simulink model "FlameAnalysis"  (R2015b)
settings: Solver=ode45  SolverMode=SingleTasking  StartTime=0.0  StopTime=1000  RelTol=1e-3
PreLoadFcn:
  | fprintf('loading now...\n')
PostLoadFcn:
  | model_name = gcs;
  | video_player_name=[model_name, '/From Multimedia File'];
  | video_path=get_param(video_player_name,'inputFileName');
  | model_path= get_param(model_name,'filename');
  | i=findstr('\',model_path);
  | 
  | if(~exist(video_path))
  |      video_path2=[model_path(1:i(end))  video_path(findstr('Video',video_path):end)];
  | 
  |      if(exist(video_path2))
  |           set_param(video_player_name,'inputFileName',video_path2);
  |      else
  |           j=findstr('\',video_path);
  |           video_path2=[model_path(1:i(end))  'Videos\' video_path(j(end)+1:end)];
  |           if(exist(video_path2))
  |                set_param(video_player_name,'inputFileName',video_path2);
  |           else
  |                avifiles=dir('videos\*.avi')
  |                set_param(video_player_name,'inputFileName',[model_path(1:i(end))  'Videos\'   avifiles(1).name]);
  |           end
  | 
  |      end
  | end
InitFcn:
  | clc
  | clear
  | global  t position wide dz_dt d2z_dt2 d3z_dt3 Af As dA_dt filePath Su_ Su alfa Karlovitz threshold model_name bords tWalls sheet model_path simulating numPointsAnalysis
  | simulating=true;
  | model_name = gcs;
  | model_path = [model_name, '/Edit Parameters'];
  | tbf = str2num(get_param(model_path,'tbf'));
  | ppcm= str2num(get_param(model_path,'ppcm'));
  | p2e= str2num(get_param(model_path,'p2e'));
  | 
  | nframes0= str2num(get_param(model_path,'nframes0'));
  | alfa= str2num(get_param(model_path,'alfa'));
  | fff= str2num(get_param(model_path,'fff'));
  | 
  | if((size(fff,2)~=1) & (size(fff,2)~=2))
  |     error('The flame front fraction must be scalar or 1x2-array');
  | end
  | order=str2num(get_param(model_path,'order'));
  | numberOfPoints=str2num(get_param(model_path,'numberOfPoints'));
  | orderAnalysis=str2num(get_param(model_path,'orderAnalysis'));
  | numPointsAnalysis=str2num(get_param(model_path,'numPointsAnalysis'));
  | uselog=str2num(get_param(model_path,'uselog'));
  | 
  | 
  | save2xls= strcmp('on',get_param(model_path,'save2xls'));
  | saveVideo= strcmp('on',get_param(model_path,'saveVideo'));
  | cfs= strcmp('on',get_param(model_path,'cfs'));
  | c3dv= strcmp('on',get_param(model_path,'c3dv'));
  | 
  | 
  | if(strcmp(get_param(model_path,'bge'),'Temporal Median Estimator'))
  |      bge=1;
  | elseif (strcmp(get_param(model_path,'bge'),'Temporal Median'))
  |     bge=2;
  |     bkgnd{1}=[gcs '/Background Estimator/Decomposing Red Movement/BG1/Temporal Median/Temporal Median'];
  |     bkgnd{2}=[gcs '/Background Estimator/Decomposing Green Movement/BG1/Temporal Median/Temporal Median'];
  |     bkgnd{3}=[gcs '/Background Estimator/Decomposing Blue Movement/BG1/Temporal Median/Temporal Median'];
  | 
  |     nframes0=max(nframes0,1);
  |     set_param([gcs '/Edit Parameters/'],'nframes0',num2str(nframes0));
  |     for i=1:3
  |         set_param(bkgnd{i}, 'tw', num2str(nframes0));
  |     end
  | else
  |     bge=3;
  | end
  | 
  | 
  | 
  | switch(get_param(model_path,'aprox_type'))
  |      case 'Profile'
  |            aprox_type=1;
  |            sheet='Profile';
  |      case 'Paraboloid (moving base)'
  |            aprox_type=2;
  |            sheet='Paraboloid';
  |      case 'Paraboloid(fixed base)'
  |            aprox_type=3;
  |            sheet='ParaboloidFB';
  |      case 'Spheroid'
  | ... (+19 lines)
StopFcn:
  | global editing  simulating
  | simulating = true;
  | try
  |       closeFunction
  | catch err
  |       simulating=false;
  |       err
  | end
  |   simulating=false;
model workspace (MATLAB code in the model file):
  | line_row =  22;
values from neighbouring files (symbols this model uses):
  m = size(BW,1)    [flameFront.m]    (also in putCircles.m = (y(i+1)-y(i))./(x(i+1)-x(i)))
  n = n(n==size(num,2)/4)    [averageOfVideos.m]    (also in countFramesOfVideo.m = 1; putCircles.m = length(y))
  vector = cast([row, col],'double')    [flameFront.m]
undefined symbols (not defined in the file or in its folder): strel
libraries: simulink x27, visionstatistics x14, visionconversions x9, visiontextngfix x9, visionmorphops x7, dspvision x4, visionsinks x2, visiongeotforms x1
(part 2 of 3)

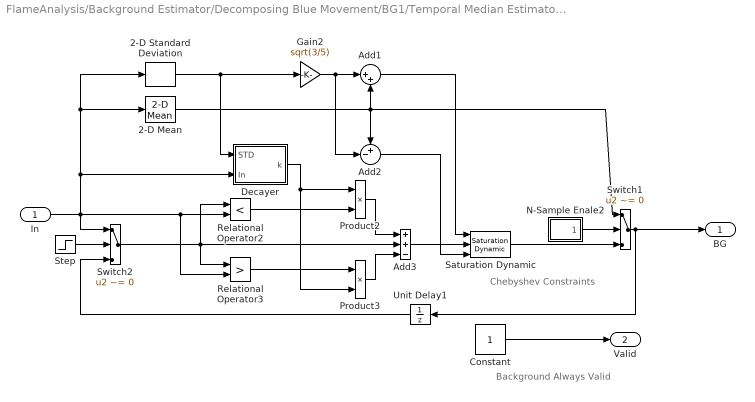
== system FlameAnalysis/Background Estimator/Decomposing Blue Movement/BG1/Temporal Median Estimator/Temporal Median Estimator ==
  note: Background
      | Always Valid
  note: Chebyshev
      | Constraints
  In : Inport
  2-D Mean : visionstatistics/2-D Mean  run=on  reset_popup=None  directionMode=Entire input  dimension=1  treatSBRowAsCol=on  roiEnable=off  roiType=Rectangles  roiPortion=Entire ROI  roiOutput=Individual statistics for each ROI  roiFlag=off  outputDataTypeStr=Inherit: Same as accumulator  outputLastDataTypeStr=Inherit: Same as accumulator  outputMin=[]  outputMax=[]  roundingMode=Floor  overflowMode=off
  2-D Standard Deviation : visionstatistics/2-D Standard Deviation  run=on  reset_popup=None  directionMode=Entire input  dimension=1  treatSBRowAsCol=on  roiEnable=off  roiType=Rectangles  roiPortion=Entire ROI  roiOutput=Individual statistics for each ROI  roiFlag=off
  Add1 : Sum  Inputs=|++
  Add2 : Sum  Inputs=+-|
  Add3 : Sum  Inputs=++-
  Constant : Constant  OutDataTypeStr=boolean
  Decayer : Subsystem
  Gain2 : Gain  Gain=sqrt(3/5)
  N-Sample Enale2 : Subsystem  mask(N Sample Enable){sample=t0}
      mask prompts: sample "Trigger Count, N"
      mask help: Active Level = Low(0)
  Product2 : Product  RndMeth=Zero
  Product3 : Product  RndMeth=Zero
  Relational Operator2 : RelationalOperator  Operator=<  OutDataTypeStr=uint(8)
  Relational Operator3 : RelationalOperator  Operator=>  OutDataTypeStr=uint(8)
  Saturation Dynamic : simulink/Discontinuities/Saturation Dynamic  OutMin=[]  OutMax=[]  OutDataTypeStr=Inherit: Same as second input  OutDataType=fixdt(1, 16)  OutScaling=2^-10  DoSatur=off
  Step : Step  Time=eps  Before=1  After=0
  Switch1 : Switch  Criteria=u2 ~= 0
  Switch2 : Switch  Criteria=u2 ~= 0
  Unit Delay1 : UnitDelay  SampleTime=-1
  BG : Outport
  Valid : Outport  Port=2
  wires:
  Add1/1 -> Saturation Dynamic/1
  Constant/1 -> Valid/1
  Add2/1 -> Saturation Dynamic/3
  2-D Mean/1 -> Add2/1, Add1/2, Switch1/1
  Gain2/1 -> Add2/2, Add1/1
  Add3/1 -> Saturation Dynamic/2
  Step/1 -> Switch2/2
  Unit Delay1/1 -> Switch2/3
  Switch2/1 -> Add3/2, Relational Operator2/1, Relational Operator3/1
  N-Sample Enale2/1(Enable) -> Switch1/2
  Switch1/1 -> BG/1, Unit Delay1/1
  In/1 -> Switch2/1, Relational Operator2/2, Relational Operator3/2, 2-D Standard Deviation/1, 2-D Mean/1, Decayer/2(In)
  Relational Operator2/1 -> Product2/2
  Relational Operator3/1 -> Product3/1
  Saturation Dynamic/1 -> Switch1/3
  2-D Standard Deviation/1 -> Decayer/1(STD), Gain2/1
  Decayer/1(k) -> Product2/1, Product3/2
  Product2/1 -> Add3/1
  Product3/1 -> Add3/3

== system FlameAnalysis/Background Estimator/Decomposing Green Movement/BG1/Motion Based Background Estimator/Motion Based Background Estimator ==
  In : Inport
  BG_running : Subsystem
  Logical Operator : Logic  Operator=NOT
  Unit Delay : UnitDelay  SampleTime=-1
  BG : Outport
  Valid : Outport  Port=2
  wires:
  Unit Delay/1 -> Logical Operator/1
  BG_running/1(BG) -> BG/1
  In/1 -> BG_running/1(In1)
  Logical Operator/1 -> BG_running/Enable
  BG_running/2(bgflag) -> Valid/1, Unit Delay/1

== system FlameAnalysis/Background Estimator/Decomposing Green Movement/BG1/Temporal Median/Temporal Median ==
  In : Inport
  Background estimator : Subsystem  TreatAsAtomicUnit=on
  Logical Operator1 : Logic  Operator=NOT
  N-Sample Enale2 : Subsystem  mask(N Sample Enable){sample=tw}
      mask prompts: sample "Trigger Count, N"
      mask help: Active Level = Low(0)
  BG : Outport
  Valid : Outport  Port=2
  wires:
  In/1 -> Background estimator/1(Video In)
  Background estimator/1(Background) -> BG/1
  N-Sample Enale2/1(Enable) -> Background estimator/Enable, Logical Operator1/1
  Logical Operator1/1 -> Valid/1

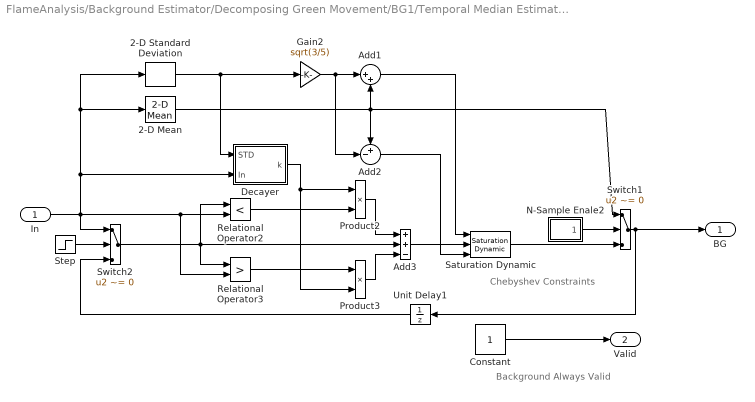
== system FlameAnalysis/Background Estimator/Decomposing Green Movement/BG1/Temporal Median Estimator/Temporal Median Estimator ==
  note: Background
      | Always Valid
  note: Chebyshev
      | Constraints
  In : Inport
  2-D Mean : visionstatistics/2-D Mean  run=on  reset_popup=None  directionMode=Entire input  dimension=1  treatSBRowAsCol=on  roiEnable=off  roiType=Rectangles  roiPortion=Entire ROI  roiOutput=Individual statistics for each ROI  roiFlag=off  outputDataTypeStr=Inherit: Same as accumulator  outputLastDataTypeStr=Inherit: Same as accumulator  outputMin=[]  outputMax=[]  roundingMode=Floor  overflowMode=off
  2-D Standard Deviation : visionstatistics/2-D Standard Deviation  run=on  reset_popup=None  directionMode=Entire input  dimension=1  treatSBRowAsCol=on  roiEnable=off  roiType=Rectangles  roiPortion=Entire ROI  roiOutput=Individual statistics for each ROI  roiFlag=off
  Add1 : Sum  Inputs=|++
  Add2 : Sum  Inputs=+-|
  Add3 : Sum  Inputs=++-
  Constant : Constant  OutDataTypeStr=boolean
  Decayer : Subsystem
  Gain2 : Gain  Gain=sqrt(3/5)
  N-Sample Enale2 : Subsystem  mask(N Sample Enable){sample=t0}
      mask prompts: sample "Trigger Count, N"
      mask help: Active Level = Low(0)
  Product2 : Product  RndMeth=Zero
  Product3 : Product  RndMeth=Zero
  Relational Operator2 : RelationalOperator  Operator=<  OutDataTypeStr=uint(8)
  Relational Operator3 : RelationalOperator  Operator=>  OutDataTypeStr=uint(8)
  Saturation Dynamic : simulink/Discontinuities/Saturation Dynamic  OutMin=[]  OutMax=[]  OutDataTypeStr=Inherit: Same as second input  OutDataType=fixdt(1, 16)  OutScaling=2^-10  DoSatur=off
  Step : Step  Time=eps  Before=1  After=0
  Switch1 : Switch  Criteria=u2 ~= 0
  Switch2 : Switch  Criteria=u2 ~= 0
  Unit Delay1 : UnitDelay  SampleTime=-1
  BG : Outport
  Valid : Outport  Port=2
  wires:
  Add1/1 -> Saturation Dynamic/1
  Constant/1 -> Valid/1
  Add2/1 -> Saturation Dynamic/3
  2-D Mean/1 -> Add2/1, Add1/2, Switch1/1
  Gain2/1 -> Add2/2, Add1/1
  Add3/1 -> Saturation Dynamic/2
  Step/1 -> Switch2/2
  Unit Delay1/1 -> Switch2/3
  Switch2/1 -> Add3/2, Relational Operator2/1, Relational Operator3/1
  N-Sample Enale2/1(Enable) -> Switch1/2
  Switch1/1 -> BG/1, Unit Delay1/1
  In/1 -> Switch2/1, Relational Operator2/2, Relational Operator3/2, 2-D Standard Deviation/1, 2-D Mean/1, Decayer/2(In)
  Relational Operator2/1 -> Product2/2
  Relational Operator3/1 -> Product3/1
  Saturation Dynamic/1 -> Switch1/3
  2-D Standard Deviation/1 -> Decayer/1(STD), Gain2/1
  Decayer/1(k) -> Product2/1, Product3/2
  Product2/1 -> Add3/1
  Product3/1 -> Add3/3

== system FlameAnalysis/Background Estimator/Decomposing Red Movement/BG1/Motion Based Background Estimator/Motion Based Background Estimator ==
  In : Inport
  BG_running : Subsystem
  Logical Operator : Logic  Operator=NOT
  Unit Delay : UnitDelay  SampleTime=-1
  BG : Outport
  Valid : Outport  Port=2
  wires:
  Unit Delay/1 -> Logical Operator/1
  BG_running/1(BG) -> BG/1
  In/1 -> BG_running/1(In1)
  Logical Operator/1 -> BG_running/Enable
  BG_running/2(bgflag) -> Valid/1, Unit Delay/1

== system FlameAnalysis/Background Estimator/Decomposing Red Movement/BG1/Temporal Median/Temporal Median ==
  In : Inport
  Background estimator : Subsystem  TreatAsAtomicUnit=on
  Logical Operator1 : Logic  Operator=NOT
  N-Sample Enale2 : Subsystem  mask(N Sample Enable){sample=tw}
      mask prompts: sample "Trigger Count, N"
      mask help: Active Level = Low(0)
  BG : Outport
  Valid : Outport  Port=2
  wires:
  In/1 -> Background estimator/1(Video In)
  Background estimator/1(Background) -> BG/1
  N-Sample Enale2/1(Enable) -> Background estimator/Enable, Logical Operator1/1
  Logical Operator1/1 -> Valid/1

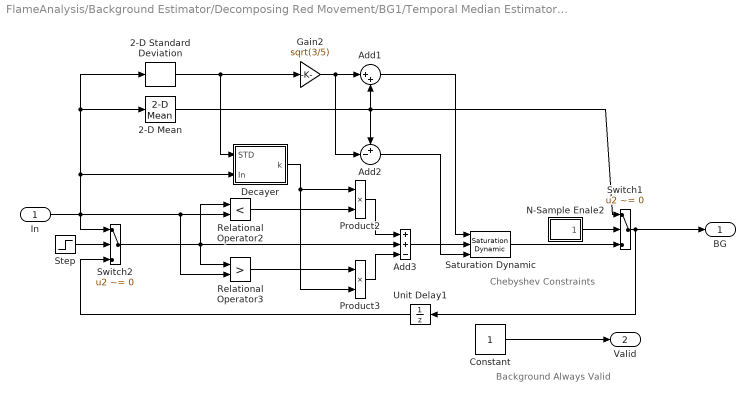
== system FlameAnalysis/Background Estimator/Decomposing Red Movement/BG1/Temporal Median Estimator/Temporal Median Estimator ==
  note: Background
      | Always Valid
  note: Chebyshev
      | Constraints
  In : Inport
  2-D Mean : visionstatistics/2-D Mean  run=on  reset_popup=None  directionMode=Entire input  dimension=1  treatSBRowAsCol=on  roiEnable=off  roiType=Rectangles  roiPortion=Entire ROI  roiOutput=Individual statistics for each ROI  roiFlag=off  outputDataTypeStr=Inherit: Same as accumulator  outputLastDataTypeStr=Inherit: Same as accumulator  outputMin=[]  outputMax=[]  roundingMode=Floor  overflowMode=off
  2-D Standard Deviation : visionstatistics/2-D Standard Deviation  run=on  reset_popup=None  directionMode=Entire input  dimension=1  treatSBRowAsCol=on  roiEnable=off  roiType=Rectangles  roiPortion=Entire ROI  roiOutput=Individual statistics for each ROI  roiFlag=off
  Add1 : Sum  Inputs=|++
  Add2 : Sum  Inputs=+-|
  Add3 : Sum  Inputs=++-
  Constant : Constant  OutDataTypeStr=boolean
  Decayer : Subsystem
  Gain2 : Gain  Gain=sqrt(3/5)
  N-Sample Enale2 : Subsystem  mask(N Sample Enable){sample=t0}
      mask prompts: sample "Trigger Count, N"
      mask help: Active Level = Low(0)
  Product2 : Product  RndMeth=Zero
  Product3 : Product  RndMeth=Zero
  Relational Operator2 : RelationalOperator  Operator=<  OutDataTypeStr=uint(8)
  Relational Operator3 : RelationalOperator  Operator=>  OutDataTypeStr=uint(8)
  Saturation Dynamic : simulink/Discontinuities/Saturation Dynamic  OutMin=[]  OutMax=[]  OutDataTypeStr=Inherit: Same as second input  OutDataType=fixdt(1, 16)  OutScaling=2^-10  DoSatur=off
  Step : Step  Time=eps  Before=1  After=0
  Switch1 : Switch  Criteria=u2 ~= 0
  Switch2 : Switch  Criteria=u2 ~= 0
  Unit Delay1 : UnitDelay  SampleTime=-1
  BG : Outport
  Valid : Outport  Port=2
  wires:
  Add1/1 -> Saturation Dynamic/1
  Constant/1 -> Valid/1
  Add2/1 -> Saturation Dynamic/3
  2-D Mean/1 -> Add2/1, Add1/2, Switch1/1
  Gain2/1 -> Add2/2, Add1/1
  Add3/1 -> Saturation Dynamic/2
  Step/1 -> Switch2/2
  Unit Delay1/1 -> Switch2/3
  Switch2/1 -> Add3/2, Relational Operator2/1, Relational Operator3/1
  N-Sample Enale2/1(Enable) -> Switch1/2
  Switch1/1 -> BG/1, Unit Delay1/1
  In/1 -> Switch2/1, Relational Operator2/2, Relational Operator3/2, 2-D Standard Deviation/1, 2-D Mean/1, Decayer/2(In)
  Relational Operator2/1 -> Product2/2
  Relational Operator3/1 -> Product3/1
  Saturation Dynamic/1 -> Switch1/3
  2-D Standard Deviation/1 -> Decayer/1(STD), Gain2/1
  Decayer/1(k) -> Product2/1, Product3/2
  Product2/1 -> Add3/1
  Product3/1 -> Add3/3

== system FlameAnalysis/Background Estimator/Decomposing Blue Movement/BG1/Motion Based Background Estimator/Motion Based Background Estimator/BG_running ==
  In1 : Inport
  Enable : EnablePort  PropagateVarSize=During execution
  CompleteBG : Subsystem
  Compositing : visiontextngfix/Compositing  operation=Binary mask  bFacSrc=Specify via dialog  mFacSrc=Input port  bFactor=0.75  mFactor=1  source=Specify via dialog  coordinates=[1 1]  prodOutputMode=Binary point scaling  prodOutputWordLength=32  prodOutputFracLength=10  roundingMode=Floor  overflowMode=off
  EvaluateFG : Subsystem
  N-Sample Enable3 : Subsystem  mask(N-Sample Enable){sample=2}
      mask prompts: sample "Trigger Count, N"
      mask help: Active = High(0)
  Switch : Switch  Criteria=u2 ~= 0
  Unit Delay : UnitDelay  SampleTime=-1
  BG : Outport
  bgflag : Outport  Port=2
  wires:
  Compositing/1 -> BG/1, Switch/1
  CompleteBG/1(fgmask) -> Compositing/3
  EvaluateFG/1(fgB) -> CompleteBG/1(fgB)
  In1/1 -> EvaluateFG/1(I), Compositing/2, Switch/3
  CompleteBG/2(bgflag) -> bgflag/1
  N-Sample Enable3/1(Enable) -> Switch/2
  Switch/1 -> Unit Delay/1
  Unit Delay/1 -> Compositing/1

== system FlameAnalysis/Background Estimator/Decomposing Blue Movement/BG1/Temporal Median/Temporal Median/Background estimator ==
  note: Estimate the background
  Video In : Inport
  Enable : EnablePort  PropagateVarSize=During execution
  2-D Median : visionstatistics/2-D Median  sortAlg=Quick sort  directionMode=Each column  dimension=1  treatSBRowAsCol=on  outputDataTypeStr=Inherit: Same as accumulator  outputLastDataTypeStr=Inherit: Same as accumulator  outputMin=[]  outputMax=[]  accumDataTypeStr=Inherit: Same as product output  accumLastDataTypeStr=Inherit: Same as product output  roundingMode=Floor  overflowMode=off
      settings: allowOverrides=off
  Buffer : Buffer  N=tw  V=tw-1  TreatMby1Signals=One channel
  Frame Conversion1 : FrameConversion  InheritSamplingMode=off  OutFrame=Sample-based
  Reshape : Reshape  OutputDimensionality=Row vector (2-D)
  Reshape1 : Reshape  OutputDimensionality=Derive from reference input port  OutputDimensions=[120 160]
  Background : Outport
  wires:
  Reshape1/1 -> Background/1
  Reshape/1 -> Buffer/1
  Video In/1 -> Reshape/1, Reshape1/2
  Frame Conversion1/1 -> Reshape1/1
  Buffer/1 -> 2-D Median/1
  2-D Median/1 -> Frame Conversion1/1

== system FlameAnalysis/Background Estimator/Decomposing Blue Movement/BG1/Temporal Median/Temporal Median/N-Sample Enale2 ==
  Constant : Constant  OutDataTypeStr=boolean
  Constant1 : Constant  Value=0  OutDataTypeStr=boolean
  Counter Limited : simulink/Sources/Counter Limited  uplimit=sample  tsamp=-1
  Enabled Subsystem : Subsystem  TreatAsAtomicUnit=on
  Switch : Switch  Threshold=sample
  Enable : Outport
  wires:
  Enabled Subsystem/1(Out1) -> Enable/1
  Switch/1 -> Enabled Subsystem/Enable
  Constant/1 -> Switch/1
  Constant1/1 -> Switch/3
  Counter Limited/1 -> Switch/2

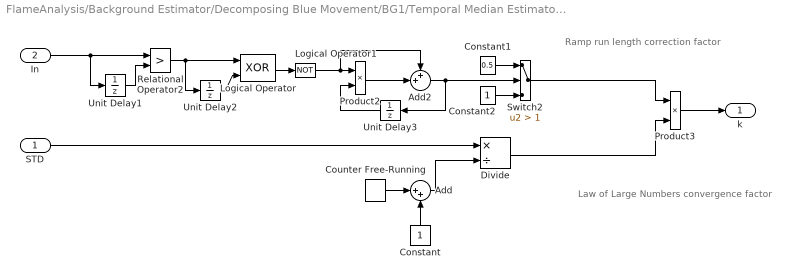
== system FlameAnalysis/Background Estimator/Decomposing Blue Movement/BG1/Temporal Median Estimator/Temporal Median Estimator/Decayer ==
  note: Ramp run length correction factor
  note: Law of Large Numbers convergence factor
  STD : Inport
  In : Inport  Port=2
  Add : Sum  Inputs=|++
  Add2 : Sum  Inputs=++|  OutDataTypeStr=single
  Constant : Constant  OutDataTypeStr=single
  Constant1 : Constant  Value=0.5  OutDataTypeStr=Inherit: Inherit via back propagation
  Constant2 : Constant  OutDataTypeStr=Inherit: Inherit via back propagation
  Counter Free-Running : simulink/Sources/Counter Free-Running  NumBits=16  tsamp=-1
  Divide : Product  Inputs=*/  OutDataTypeStr=single
  Logical Operator : Logic  Operator=XOR  AllPortsSameDT=off  OutDataTypeStr=boolean
  Logical Operator1 : Logic  Operator=NOT  AllPortsSameDT=off  OutDataTypeStr=boolean
  Product2 : Product  RndMeth=Zero
  Product3 : Product  RndMeth=Zero
  Relational Operator2 : RelationalOperator  Operator=>  OutDataTypeStr=boolean
  Switch2 : Switch  Criteria=u2 > Threshold  Threshold=1
  Unit Delay1 : UnitDelay  SampleTime=-1
  Unit Delay2 : UnitDelay  InitialCondition=1  SampleTime=-1
  Unit Delay3 : UnitDelay  SampleTime=-1
  k : Outport
  wires:
  Constant/1 -> Add/2
  Constant1/1 -> Switch2/1
  Constant2/1 -> Switch2/3
  Product3/1 -> k/1
  In/1 -> Unit Delay1/1, Relational Operator2/1
  Unit Delay3/1 -> Product2/2
  Add2/1 -> Switch2/2, Unit Delay3/1
  Product2/1 -> Add2/2
  Logical Operator1/1 -> Product2/1, Add2/1
  Logical Operator/1 -> Logical Operator1/1
  Unit Delay2/1 -> Logical Operator/2
  Relational Operator2/1 -> Unit Delay2/1, Logical Operator/1
  Unit Delay1/1 -> Relational Operator2/2
  STD/1 -> Divide/1
  Counter Free-Running/1 -> Add/1
  Add/1 -> Divide/2
  Divide/1 -> Product3/2
  Switch2/1 -> Product3/1

== system FlameAnalysis/Background Estimator/Decomposing Blue Movement/BG1/Temporal Median Estimator/Temporal Median Estimator/N-Sample Enale2 ==
  Constant : Constant  OutDataTypeStr=boolean
  Constant1 : Constant  Value=0  OutDataTypeStr=boolean
  Counter Limited : simulink/Sources/Counter Limited  uplimit=sample  tsamp=-1
  Enabled Subsystem : Subsystem  TreatAsAtomicUnit=on
  Switch : Switch  Threshold=sample
  Enable : Outport
  wires:
  Enabled Subsystem/1(Out1) -> Enable/1
  Switch/1 -> Enabled Subsystem/Enable
  Constant/1 -> Switch/1
  Constant1/1 -> Switch/3
  Counter Limited/1 -> Switch/2

== system FlameAnalysis/Background Estimator/Decomposing Green Movement/BG1/Motion Based Background Estimator/Motion Based Background Estimator/BG_running ==
  In1 : Inport
  Enable : EnablePort  PropagateVarSize=During execution
  CompleteBG : Subsystem
  Compositing : visiontextngfix/Compositing  operation=Binary mask  bFacSrc=Specify via dialog  mFacSrc=Input port  bFactor=0.75  mFactor=1  source=Specify via dialog  coordinates=[1 1]  prodOutputMode=Binary point scaling  prodOutputWordLength=32  prodOutputFracLength=10  roundingMode=Floor  overflowMode=off
  EvaluateFG : Subsystem
  N-Sample Enable3 : Subsystem  mask(N-Sample Enable){sample=2}
      mask prompts: sample "Trigger Count, N"
      mask help: Active = High(0)
  Switch : Switch  Criteria=u2 ~= 0
  Unit Delay : UnitDelay  SampleTime=-1
  BG : Outport
  bgflag : Outport  Port=2
  wires:
  Compositing/1 -> BG/1, Switch/1
  CompleteBG/1(fgmask) -> Compositing/3
  EvaluateFG/1(fgB) -> CompleteBG/1(fgB)
  In1/1 -> EvaluateFG/1(I), Compositing/2, Switch/3
  CompleteBG/2(bgflag) -> bgflag/1
  N-Sample Enable3/1(Enable) -> Switch/2
  Switch/1 -> Unit Delay/1
  Unit Delay/1 -> Compositing/1

== system FlameAnalysis/Background Estimator/Decomposing Green Movement/BG1/Temporal Median/Temporal Median/Background estimator ==
  note: Estimate the background
  Video In : Inport
  Enable : EnablePort  PropagateVarSize=During execution
  2-D Median : visionstatistics/2-D Median  sortAlg=Quick sort  directionMode=Each column  dimension=1  treatSBRowAsCol=on  outputDataTypeStr=Inherit: Same as accumulator  outputLastDataTypeStr=Inherit: Same as accumulator  outputMin=[]  outputMax=[]  accumDataTypeStr=Inherit: Same as product output  accumLastDataTypeStr=Inherit: Same as product output  roundingMode=Floor  overflowMode=off
      settings: allowOverrides=off
  Buffer : Buffer  N=tw  V=tw-1  TreatMby1Signals=One channel
  Frame Conversion1 : FrameConversion  InheritSamplingMode=off  OutFrame=Sample-based
  Reshape : Reshape  OutputDimensionality=Row vector (2-D)
  Reshape1 : Reshape  OutputDimensionality=Derive from reference input port  OutputDimensions=[120 160]
  Background : Outport
  wires:
  Reshape1/1 -> Background/1
  Reshape/1 -> Buffer/1
  Video In/1 -> Reshape/1, Reshape1/2
  Frame Conversion1/1 -> Reshape1/1
  Buffer/1 -> 2-D Median/1
  2-D Median/1 -> Frame Conversion1/1

== system FlameAnalysis/Background Estimator/Decomposing Green Movement/BG1/Temporal Median/Temporal Median/N-Sample Enale2 ==
  Constant : Constant  OutDataTypeStr=boolean
  Constant1 : Constant  Value=0  OutDataTypeStr=boolean
  Counter Limited : simulink/Sources/Counter Limited  uplimit=sample  tsamp=-1
  Enabled Subsystem : Subsystem  TreatAsAtomicUnit=on
  Switch : Switch  Threshold=sample
  Enable : Outport
  wires:
  Enabled Subsystem/1(Out1) -> Enable/1
  Switch/1 -> Enabled Subsystem/Enable
  Constant/1 -> Switch/1
  Constant1/1 -> Switch/3
  Counter Limited/1 -> Switch/2

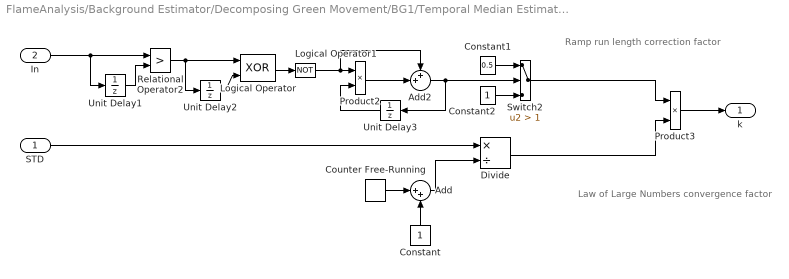
== system FlameAnalysis/Background Estimator/Decomposing Green Movement/BG1/Temporal Median Estimator/Temporal Median Estimator/Decayer ==
  note: Ramp run length correction factor
  note: Law of Large Numbers convergence factor
  STD : Inport
  In : Inport  Port=2
  Add : Sum  Inputs=|++
  Add2 : Sum  Inputs=++|  OutDataTypeStr=single
  Constant : Constant  OutDataTypeStr=single
  Constant1 : Constant  Value=0.5  OutDataTypeStr=Inherit: Inherit via back propagation
  Constant2 : Constant  OutDataTypeStr=Inherit: Inherit via back propagation
  Counter Free-Running : simulink/Sources/Counter Free-Running  NumBits=16  tsamp=-1
  Divide : Product  Inputs=*/  OutDataTypeStr=single
  Logical Operator : Logic  Operator=XOR  AllPortsSameDT=off  OutDataTypeStr=boolean
  Logical Operator1 : Logic  Operator=NOT  AllPortsSameDT=off  OutDataTypeStr=boolean
  Product2 : Product  RndMeth=Zero
  Product3 : Product  RndMeth=Zero
  Relational Operator2 : RelationalOperator  Operator=>  OutDataTypeStr=boolean
  Switch2 : Switch  Criteria=u2 > Threshold  Threshold=1
  Unit Delay1 : UnitDelay  SampleTime=-1
  Unit Delay2 : UnitDelay  InitialCondition=1  SampleTime=-1
  Unit Delay3 : UnitDelay  SampleTime=-1
  k : Outport
  wires:
  Constant/1 -> Add/2
  Constant1/1 -> Switch2/1
  Constant2/1 -> Switch2/3
  Product3/1 -> k/1
  In/1 -> Unit Delay1/1, Relational Operator2/1
  Unit Delay3/1 -> Product2/2
  Add2/1 -> Switch2/2, Unit Delay3/1
  Product2/1 -> Add2/2
  Logical Operator1/1 -> Product2/1, Add2/1
  Logical Operator/1 -> Logical Operator1/1
  Unit Delay2/1 -> Logical Operator/2
  Relational Operator2/1 -> Unit Delay2/1, Logical Operator/1
  Unit Delay1/1 -> Relational Operator2/2
  STD/1 -> Divide/1
  Counter Free-Running/1 -> Add/1
  Add/1 -> Divide/2
  Divide/1 -> Product3/2
  Switch2/1 -> Product3/1

== system FlameAnalysis/Background Estimator/Decomposing Green Movement/BG1/Temporal Median Estimator/Temporal Median Estimator/N-Sample Enale2 ==
  Constant : Constant  OutDataTypeStr=boolean
  Constant1 : Constant  Value=0  OutDataTypeStr=boolean
  Counter Limited : simulink/Sources/Counter Limited  uplimit=sample  tsamp=-1
  Enabled Subsystem : Subsystem  TreatAsAtomicUnit=on
  Switch : Switch  Threshold=sample
  Enable : Outport
  wires:
  Enabled Subsystem/1(Out1) -> Enable/1
  Switch/1 -> Enabled Subsystem/Enable
  Constant/1 -> Switch/1
  Constant1/1 -> Switch/3
  Counter Limited/1 -> Switch/2

== system FlameAnalysis/Background Estimator/Decomposing Red Movement/BG1/Motion Based Background Estimator/Motion Based Background Estimator/BG_running ==
  In1 : Inport
  Enable : EnablePort  PropagateVarSize=During execution
  CompleteBG : Subsystem
  Compositing : visiontextngfix/Compositing  operation=Binary mask  bFacSrc=Specify via dialog  mFacSrc=Input port  bFactor=0.75  mFactor=1  source=Specify via dialog  coordinates=[1 1]  prodOutputMode=Binary point scaling  prodOutputWordLength=32  prodOutputFracLength=10  roundingMode=Floor  overflowMode=off
  EvaluateFG : Subsystem
  N-Sample Enable3 : Subsystem  mask(N-Sample Enable){sample=2}
      mask prompts: sample "Trigger Count, N"
      mask help: Active = High(0)
  Switch : Switch  Criteria=u2 ~= 0
  Unit Delay : UnitDelay  SampleTime=-1
  BG : Outport
  bgflag : Outport  Port=2
  wires:
  Compositing/1 -> BG/1, Switch/1
  CompleteBG/1(fgmask) -> Compositing/3
  EvaluateFG/1(fgB) -> CompleteBG/1(fgB)
  In1/1 -> EvaluateFG/1(I), Compositing/2, Switch/3
  CompleteBG/2(bgflag) -> bgflag/1
  N-Sample Enable3/1(Enable) -> Switch/2
  Switch/1 -> Unit Delay/1
  Unit Delay/1 -> Compositing/1

== system FlameAnalysis/Background Estimator/Decomposing Red Movement/BG1/Temporal Median/Temporal Median/Background estimator ==
  note: Estimate the background
  Video In : Inport
  Enable : EnablePort  PropagateVarSize=During execution
  2-D Median : visionstatistics/2-D Median  sortAlg=Quick sort  directionMode=Each column  dimension=1  treatSBRowAsCol=on  outputDataTypeStr=Inherit: Same as accumulator  outputLastDataTypeStr=Inherit: Same as accumulator  outputMin=[]  outputMax=[]  accumDataTypeStr=Inherit: Same as product output  accumLastDataTypeStr=Inherit: Same as product output  roundingMode=Floor  overflowMode=off
      settings: allowOverrides=off
  Buffer : Buffer  N=tw  V=tw-1  TreatMby1Signals=One channel
  Frame Conversion1 : FrameConversion  InheritSamplingMode=off  OutFrame=Sample-based
  Reshape : Reshape  OutputDimensionality=Row vector (2-D)
  Reshape1 : Reshape  OutputDimensionality=Derive from reference input port  OutputDimensions=[120 160]
  Background : Outport
  wires:
  Reshape1/1 -> Background/1
  Reshape/1 -> Buffer/1
  Video In/1 -> Reshape/1, Reshape1/2
  Frame Conversion1/1 -> Reshape1/1
  Buffer/1 -> 2-D Median/1
  2-D Median/1 -> Frame Conversion1/1

== system FlameAnalysis/Background Estimator/Decomposing Red Movement/BG1/Temporal Median/Temporal Median/N-Sample Enale2 ==
  Constant : Constant  OutDataTypeStr=boolean
  Constant1 : Constant  Value=0  OutDataTypeStr=boolean
  Counter Limited : simulink/Sources/Counter Limited  uplimit=sample  tsamp=-1
  Enabled Subsystem : Subsystem  TreatAsAtomicUnit=on
  Switch : Switch  Threshold=sample
  Enable : Outport
  wires:
  Enabled Subsystem/1(Out1) -> Enable/1
  Switch/1 -> Enabled Subsystem/Enable
  Constant/1 -> Switch/1
  Constant1/1 -> Switch/3
  Counter Limited/1 -> Switch/2

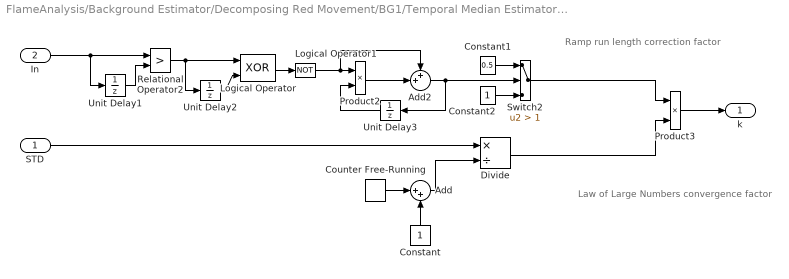
== system FlameAnalysis/Background Estimator/Decomposing Red Movement/BG1/Temporal Median Estimator/Temporal Median Estimator/Decayer ==
  note: Ramp run length correction factor
  note: Law of Large Numbers convergence factor
  STD : Inport
  In : Inport  Port=2
  Add : Sum  Inputs=|++
  Add2 : Sum  Inputs=++|  OutDataTypeStr=single
  Constant : Constant  OutDataTypeStr=single
  Constant1 : Constant  Value=0.5  OutDataTypeStr=Inherit: Inherit via back propagation
  Constant2 : Constant  OutDataTypeStr=Inherit: Inherit via back propagation
  Counter Free-Running : simulink/Sources/Counter Free-Running  NumBits=16  tsamp=-1
  Divide : Product  Inputs=*/  OutDataTypeStr=single
  Logical Operator : Logic  Operator=XOR  AllPortsSameDT=off  OutDataTypeStr=boolean
  Logical Operator1 : Logic  Operator=NOT  AllPortsSameDT=off  OutDataTypeStr=boolean
  Product2 : Product  RndMeth=Zero
  Product3 : Product  RndMeth=Zero
  Relational Operator2 : RelationalOperator  Operator=>  OutDataTypeStr=boolean
  Switch2 : Switch  Criteria=u2 > Threshold  Threshold=1
  Unit Delay1 : UnitDelay  SampleTime=-1
  Unit Delay2 : UnitDelay  InitialCondition=1  SampleTime=-1
  Unit Delay3 : UnitDelay  SampleTime=-1
  k : Outport
  wires:
  Constant/1 -> Add/2
  Constant1/1 -> Switch2/1
  Constant2/1 -> Switch2/3
  Product3/1 -> k/1
  In/1 -> Unit Delay1/1, Relational Operator2/1
  Unit Delay3/1 -> Product2/2
  Add2/1 -> Switch2/2, Unit Delay3/1
  Product2/1 -> Add2/2
  Logical Operator1/1 -> Product2/1, Add2/1
  Logical Operator/1 -> Logical Operator1/1
  Unit Delay2/1 -> Logical Operator/2
  Relational Operator2/1 -> Unit Delay2/1, Logical Operator/1
  Unit Delay1/1 -> Relational Operator2/2
  STD/1 -> Divide/1
  Counter Free-Running/1 -> Add/1
  Add/1 -> Divide/2
  Divide/1 -> Product3/2
  Switch2/1 -> Product3/1

== system FlameAnalysis/Background Estimator/Decomposing Red Movement/BG1/Temporal Median Estimator/Temporal Median Estimator/N-Sample Enale2 ==
  Constant : Constant  OutDataTypeStr=boolean
  Constant1 : Constant  Value=0  OutDataTypeStr=boolean
  Counter Limited : simulink/Sources/Counter Limited  uplimit=sample  tsamp=-1
  Enabled Subsystem : Subsystem  TreatAsAtomicUnit=on
  Switch : Switch  Threshold=sample
  Enable : Outport
  wires:
  Enabled Subsystem/1(Out1) -> Enable/1
  Switch/1 -> Enabled Subsystem/Enable
  Constant/1 -> Switch/1
  Constant1/1 -> Switch/3
  Counter Limited/1 -> Switch/2

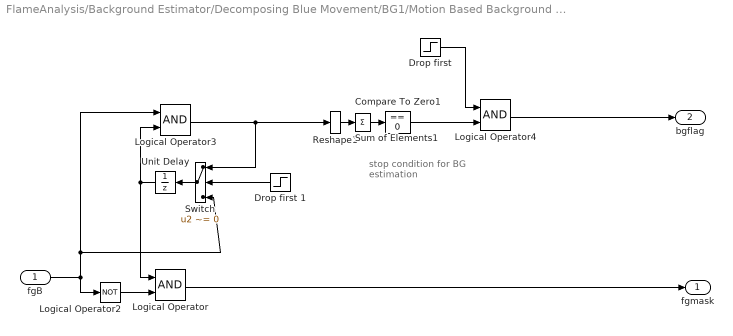
== system FlameAnalysis/Background Estimator/Decomposing Blue Movement/BG1/Motion Based Background Estimator/Motion Based Background Estimator/BG_running/CompleteBG ==
  note: stop condition
      | for BG estimation
  fgB : Inport
  Compare To Zero1 : simulink/Logic and Bit Operations/Compare To Zero  relop===  OutDataTypeStr=uint8  ZeroCross=off
  Drop first : Step  Time=eps
  Drop first 1 : Step  Time=eps
  Logical Operator : Logic  AllPortsSameDT=off  OutDataTypeStr=boolean
  Logical Operator2 : Logic  Operator=NOT  AllPortsSameDT=off  OutDataTypeStr=boolean
  Logical Operator3 : Logic  AllPortsSameDT=off  OutDataTypeStr=boolean
  Logical Operator4 : Logic  AllPortsSameDT=off  OutDataTypeStr=boolean
  Reshape1 : Reshape
  Sum of Elements1 : Sum  Inputs=+
  Switch : Switch  Criteria=u2 ~= 0
  Unit Delay : UnitDelay  SampleTime=-1
  fgmask : Outport
  bgflag : Outport  Port=2
  wires:
  fgB/1 -> Switch/3, Logical Operator3/1, Logical Operator2/1
  Logical Operator/1 -> fgmask/1
  Drop first 1/1 -> Switch/2
  Switch/1 -> Unit Delay/1
  Unit Delay/1 -> Logical Operator/1, Logical Operator3/2
  Compare To Zero1/1 -> Logical Operator4/2
  Logical Operator4/1 -> bgflag/1
  Drop first/1 -> Logical Operator4/1
  Sum of Elements1/1 -> Compare To Zero1/1
  Logical Operator3/1 -> Reshape1/1, Switch/1
  Reshape1/1 -> Sum of Elements1/1
  Logical Operator2/1 -> Logical Operator/2

== system FlameAnalysis/Background Estimator/Decomposing Blue Movement/BG1/Motion Based Background Estimator/Motion Based Background Estimator/BG_running/EvaluateFG ==
  note: detect motion for foreground
  I : Inport
  Abs3 : Abs  SaturateOnIntegerOverflow=on
  Add : Sum  Inputs=+-
  Autothreshold1 : visionconversions/Autothreshold  operator=>  threshOut=off  effMetricOut=off  userDefinedRange=off  umin=0  umax=255  outOfRngOpt=Warn and saturate  scaleThreshold=off  scaleFactor=1  P1Mode=Specify word length  P1WordLength=32  P1FracLength=30  P2Mode=Specify word length  P2WordLength=32  P2FracLength=22  P3Mode=Specify word length  P3WordLength=32  P3FracLength=14  P4Mode=Binary point scaling  P4WordLength=32  P4FracLength=15  Q1Mode=Specify word length  Q1WordLength=32  Q1FracLength=16  EMMode=Specify word length  EMWordLength=16  EMFracLength=14  roundingMode=Floor  overflowMode=off
  Blob Analysis : visionstatistics/Blob Analysis  Tag=vipblks_row_conv  area=off  centroid=off  bBox=on  majorAxis=off  minorAxis=off  angle=off  eccentricity=off  equivDiameterSq=off  extent=off  perimeter=off  maxBlobs=50  warnIfNumBlobsExceeded=on  isCount=off  useMinArea=off  minArea=0  useMaxArea=off  maxArea=inf  excludeBorderBlob=off  outDT=double  isOutVarDim=off  isFill=on  fillValues=-1  conn=8  isLabel=off  outputMode=Binary point scaling  outputWordLength=32  outputFracLength=16  firstCoeffMode=Binary point scaling  firstCoeffWordLength=16  firstCoeffFracLength=14  secondCoeffMode=Binary point scaling  secondCoeffWordLength=32  secondCoeffFracLength=16  accumMode=Binary point scaling  accumWordLength=32  accumFracLength=0  prodOutputMode=Binary point scaling  prodOutputWordLength=32  prodOutputFracLength=16  roundingMode=Floor  overflowMode=off
  BoxForeground : visiontextngfix/Draw Shapes  shape=Rectangles  fill=on  lineWidth=1  fillClrSource=Specify via dialog  display=White  intensity=200  color=[0 1 0]  opacity=1  viewport=Entire image  antialiasing=off  inType=Intensity  imagePorts=One multidimensional signal  prodOutputMode=Binary point scaling  prodOutputWordLength=32  prodOutputFracLength=14  memoryMode=Specify word length  memoryWordLength=16  memoryFracLength=15  roundingMode=Floor  overflowMode=off
  Closing : visionmorphops/Closing  nhoodsrc=Specify via dialog  strel=strel('square',5)
  Dilation : visionmorphops/Dilation  nhoodsrc=Specify via dialog  strel=[1 1 1; 1 1 1; 1 1 1]
  Manual Switch : ManualSwitch
  Unit Delay : UnitDelay  SampleTime=-1
  fgB : Outport
  wires:
  Unit Delay/1 -> Add/1
  I/1 -> Add/2, Unit Delay/1
  Autothreshold1/1 -> Closing/1
  Add/1 -> Abs3/1
  Abs3/1 -> Autothreshold1/1
  Blob Analysis/1 -> BoxForeground/2
  Closing/1 -> Dilation/1
  Dilation/1 -> BoxForeground/1, Blob Analysis/1, Manual Switch/2
  Manual Switch/1 -> fgB/1
  BoxForeground/1 -> Manual Switch/1

== system FlameAnalysis/Background Estimator/Decomposing Blue Movement/BG1/Motion Based Background Estimator/Motion Based Background Estimator/BG_running/N-Sample Enable3 ==
  Constant : Constant  OutDataTypeStr=boolean
  Constant1 : Constant  Value=0  OutDataTypeStr=boolean
  Counter Limited : simulink/Sources/Counter Limited  uplimit=sample  tsamp=-1
  Enabled Subsystem : Subsystem  TreatAsAtomicUnit=on
  Switch : Switch  Threshold=sample
  Enable : Outport
  wires:
  Counter Limited/1 -> Switch/2
  Constant1/1 -> Switch/3
  Constant/1 -> Switch/1
  Switch/1 -> Enabled Subsystem/Enable
  Enabled Subsystem/1(Out1) -> Enable/1

== system FlameAnalysis/Background Estimator/Decomposing Blue Movement/BG1/Temporal Median/Temporal Median/N-Sample Enale2/Enabled Subsystem ==
  Enable : EnablePort
  Constant : Constant  Value=0  OutDataTypeStr=boolean
  Out1 : Outport  InitialOutput=1
  wires:
  Constant/1 -> Out1/1

== system FlameAnalysis/Background Estimator/Decomposing Blue Movement/BG1/Temporal Median Estimator/Temporal Median Estimator/N-Sample Enale2/Enabled Subsystem ==
  Enable : EnablePort
  Constant : Constant  Value=0  OutDataTypeStr=boolean
  Out1 : Outport  InitialOutput=1
  wires:
  Constant/1 -> Out1/1

== system FlameAnalysis/Background Estimator/Decomposing Green Movement/BG1/Motion Based Background Estimator/Motion Based Background Estimator/BG_running/CompleteBG ==
  note: stop condition
      | for BG estimation
  fgB : Inport
  Compare To Zero1 : simulink/Logic and Bit Operations/Compare To Zero  relop===  OutDataTypeStr=uint8  ZeroCross=off
  Drop first : Step  Time=eps
  Drop first 1 : Step  Time=eps
  Logical Operator : Logic  AllPortsSameDT=off  OutDataTypeStr=boolean
  Logical Operator2 : Logic  Operator=NOT  AllPortsSameDT=off  OutDataTypeStr=boolean
  Logical Operator3 : Logic  AllPortsSameDT=off  OutDataTypeStr=boolean
  Logical Operator4 : Logic  AllPortsSameDT=off  OutDataTypeStr=boolean
  Reshape1 : Reshape
  Sum of Elements1 : Sum  Inputs=+
  Switch : Switch  Criteria=u2 ~= 0
  Unit Delay : UnitDelay  SampleTime=-1
  fgmask : Outport
  bgflag : Outport  Port=2
  wires:
  fgB/1 -> Switch/3, Logical Operator3/1, Logical Operator2/1
  Logical Operator/1 -> fgmask/1
  Drop first 1/1 -> Switch/2
  Switch/1 -> Unit Delay/1
  Unit Delay/1 -> Logical Operator/1, Logical Operator3/2
  Compare To Zero1/1 -> Logical Operator4/2
  Logical Operator4/1 -> bgflag/1
  Drop first/1 -> Logical Operator4/1
  Sum of Elements1/1 -> Compare To Zero1/1
  Logical Operator3/1 -> Reshape1/1, Switch/1
  Reshape1/1 -> Sum of Elements1/1
  Logical Operator2/1 -> Logical Operator/2

== system FlameAnalysis/Background Estimator/Decomposing Green Movement/BG1/Motion Based Background Estimator/Motion Based Background Estimator/BG_running/EvaluateFG ==
  note: detect motion for foreground
  I : Inport
  Abs3 : Abs  SaturateOnIntegerOverflow=on
  Add : Sum  Inputs=+-
  Autothreshold1 : visionconversions/Autothreshold  operator=>  threshOut=off  effMetricOut=off  userDefinedRange=off  umin=0  umax=255  outOfRngOpt=Warn and saturate  scaleThreshold=off  scaleFactor=1  P1Mode=Specify word length  P1WordLength=32  P1FracLength=30  P2Mode=Specify word length  P2WordLength=32  P2FracLength=22  P3Mode=Specify word length  P3WordLength=32  P3FracLength=14  P4Mode=Binary point scaling  P4WordLength=32  P4FracLength=15  Q1Mode=Specify word length  Q1WordLength=32  Q1FracLength=16  EMMode=Specify word length  EMWordLength=16  EMFracLength=14  roundingMode=Floor  overflowMode=off
  Blob Analysis : visionstatistics/Blob Analysis  Tag=vipblks_row_conv  area=off  centroid=off  bBox=on  majorAxis=off  minorAxis=off  angle=off  eccentricity=off  equivDiameterSq=off  extent=off  perimeter=off  maxBlobs=50  warnIfNumBlobsExceeded=on  isCount=off  useMinArea=off  minArea=0  useMaxArea=off  maxArea=inf  excludeBorderBlob=off  outDT=double  isOutVarDim=off  isFill=on  fillValues=-1  conn=8  isLabel=off  outputMode=Binary point scaling  outputWordLength=32  outputFracLength=16  firstCoeffMode=Binary point scaling  firstCoeffWordLength=16  firstCoeffFracLength=14  secondCoeffMode=Binary point scaling  secondCoeffWordLength=32  secondCoeffFracLength=16  accumMode=Binary point scaling  accumWordLength=32  accumFracLength=0  prodOutputMode=Binary point scaling  prodOutputWordLength=32  prodOutputFracLength=16  roundingMode=Floor  overflowMode=off
  BoxForeground : visiontextngfix/Draw Shapes  shape=Rectangles  fill=on  lineWidth=1  fillClrSource=Specify via dialog  display=White  intensity=200  color=[0 1 0]  opacity=1  viewport=Entire image  antialiasing=off  inType=Intensity  imagePorts=One multidimensional signal  prodOutputMode=Binary point scaling  prodOutputWordLength=32  prodOutputFracLength=14  memoryMode=Specify word length  memoryWordLength=16  memoryFracLength=15  roundingMode=Floor  overflowMode=off
  Closing : visionmorphops/Closing  nhoodsrc=Specify via dialog  strel=strel('square',5)
  Dilation : visionmorphops/Dilation  nhoodsrc=Specify via dialog  strel=[1 1 1; 1 1 1; 1 1 1]
  Manual Switch : ManualSwitch
  Unit Delay : UnitDelay  SampleTime=-1
  fgB : Outport
  wires:
  Unit Delay/1 -> Add/1
  I/1 -> Add/2, Unit Delay/1
  Autothreshold1/1 -> Closing/1
  Add/1 -> Abs3/1
  Abs3/1 -> Autothreshold1/1
  Blob Analysis/1 -> BoxForeground/2
  Closing/1 -> Dilation/1
  Dilation/1 -> BoxForeground/1, Blob Analysis/1, Manual Switch/2
  Manual Switch/1 -> fgB/1
  BoxForeground/1 -> Manual Switch/1

== system FlameAnalysis/Background Estimator/Decomposing Green Movement/BG1/Motion Based Background Estimator/Motion Based Background Estimator/BG_running/N-Sample Enable3 ==
  Constant : Constant  OutDataTypeStr=boolean
  Constant1 : Constant  Value=0  OutDataTypeStr=boolean
  Counter Limited : simulink/Sources/Counter Limited  uplimit=sample  tsamp=-1
  Enabled Subsystem : Subsystem  TreatAsAtomicUnit=on
  Switch : Switch  Threshold=sample
  Enable : Outport
  wires:
  Counter Limited/1 -> Switch/2
  Constant1/1 -> Switch/3
  Constant/1 -> Switch/1
  Switch/1 -> Enabled Subsystem/Enable
  Enabled Subsystem/1(Out1) -> Enable/1

== system FlameAnalysis/Background Estimator/Decomposing Green Movement/BG1/Temporal Median/Temporal Median/N-Sample Enale2/Enabled Subsystem ==
  Enable : EnablePort
  Constant : Constant  Value=0  OutDataTypeStr=boolean
  Out1 : Outport  InitialOutput=1
  wires:
  Constant/1 -> Out1/1

== system FlameAnalysis/Background Estimator/Decomposing Green Movement/BG1/Temporal Median Estimator/Temporal Median Estimator/N-Sample Enale2/Enabled Subsystem ==
  Enable : EnablePort
  Constant : Constant  Value=0  OutDataTypeStr=boolean
  Out1 : Outport  InitialOutput=1
  wires:
  Constant/1 -> Out1/1

== system FlameAnalysis/Background Estimator/Decomposing Red Movement/BG1/Motion Based Background Estimator/Motion Based Background Estimator/BG_running/CompleteBG ==
  note: stop condition
      | for BG estimation
  fgB : Inport
  Compare To Zero1 : simulink/Logic and Bit Operations/Compare To Zero  relop===  OutDataTypeStr=uint8  ZeroCross=off
  Drop first : Step  Time=eps
  Drop first 1 : Step  Time=eps
  Logical Operator : Logic  AllPortsSameDT=off  OutDataTypeStr=boolean
  Logical Operator2 : Logic  Operator=NOT  AllPortsSameDT=off  OutDataTypeStr=boolean
  Logical Operator3 : Logic  AllPortsSameDT=off  OutDataTypeStr=boolean
  Logical Operator4 : Logic  AllPortsSameDT=off  OutDataTypeStr=boolean
  Reshape1 : Reshape
  Sum of Elements1 : Sum  Inputs=+
  Switch : Switch  Criteria=u2 ~= 0
  Unit Delay : UnitDelay  SampleTime=-1
  fgmask : Outport
  bgflag : Outport  Port=2
  wires:
  fgB/1 -> Switch/3, Logical Operator3/1, Logical Operator2/1
  Logical Operator/1 -> fgmask/1
  Drop first 1/1 -> Switch/2
  Switch/1 -> Unit Delay/1
  Unit Delay/1 -> Logical Operator/1, Logical Operator3/2
  Compare To Zero1/1 -> Logical Operator4/2
  Logical Operator4/1 -> bgflag/1
  Drop first/1 -> Logical Operator4/1
  Sum of Elements1/1 -> Compare To Zero1/1
  Logical Operator3/1 -> Reshape1/1, Switch/1
  Reshape1/1 -> Sum of Elements1/1
  Logical Operator2/1 -> Logical Operator/2

== system FlameAnalysis/Background Estimator/Decomposing Red Movement/BG1/Motion Based Background Estimator/Motion Based Background Estimator/BG_running/EvaluateFG ==
  note: detect motion for foreground
  I : Inport
  Abs3 : Abs  SaturateOnIntegerOverflow=on
  Add : Sum  Inputs=+-
  Autothreshold1 : visionconversions/Autothreshold  operator=>  threshOut=off  effMetricOut=off  userDefinedRange=off  umin=0  umax=255  outOfRngOpt=Warn and saturate  scaleThreshold=off  scaleFactor=1  P1Mode=Specify word length  P1WordLength=32  P1FracLength=30  P2Mode=Specify word length  P2WordLength=32  P2FracLength=22  P3Mode=Specify word length  P3WordLength=32  P3FracLength=14  P4Mode=Binary point scaling  P4WordLength=32  P4FracLength=15  Q1Mode=Specify word length  Q1WordLength=32  Q1FracLength=16  EMMode=Specify word length  EMWordLength=16  EMFracLength=14  roundingMode=Floor  overflowMode=off
  Blob Analysis : visionstatistics/Blob Analysis  Tag=vipblks_row_conv  area=off  centroid=off  bBox=on  majorAxis=off  minorAxis=off  angle=off  eccentricity=off  equivDiameterSq=off  extent=off  perimeter=off  maxBlobs=50  warnIfNumBlobsExceeded=on  isCount=off  useMinArea=off  minArea=0  useMaxArea=off  maxArea=inf  excludeBorderBlob=off  outDT=double  isOutVarDim=off  isFill=on  fillValues=-1  conn=8  isLabel=off  outputMode=Binary point scaling  outputWordLength=32  outputFracLength=16  firstCoeffMode=Binary point scaling  firstCoeffWordLength=16  firstCoeffFracLength=14  secondCoeffMode=Binary point scaling  secondCoeffWordLength=32  secondCoeffFracLength=16  accumMode=Binary point scaling  accumWordLength=32  accumFracLength=0  prodOutputMode=Binary point scaling  prodOutputWordLength=32  prodOutputFracLength=16  roundingMode=Floor  overflowMode=off
  BoxForeground : visiontextngfix/Draw Shapes  shape=Rectangles  fill=on  lineWidth=1  fillClrSource=Specify via dialog  display=White  intensity=200  color=[0 1 0]  opacity=1  viewport=Entire image  antialiasing=off  inType=Intensity  imagePorts=One multidimensional signal  prodOutputMode=Binary point scaling  prodOutputWordLength=32  prodOutputFracLength=14  memoryMode=Specify word length  memoryWordLength=16  memoryFracLength=15  roundingMode=Floor  overflowMode=off
  Closing : visionmorphops/Closing  nhoodsrc=Specify via dialog  strel=strel('square',5)
  Dilation : visionmorphops/Dilation  nhoodsrc=Specify via dialog  strel=[1 1 1; 1 1 1; 1 1 1]
  Manual Switch : ManualSwitch
  Unit Delay : UnitDelay  SampleTime=-1
  fgB : Outport
  wires:
  Unit Delay/1 -> Add/1
  I/1 -> Add/2, Unit Delay/1
  Autothreshold1/1 -> Closing/1
  Add/1 -> Abs3/1
  Abs3/1 -> Autothreshold1/1
  Blob Analysis/1 -> BoxForeground/2
  Closing/1 -> Dilation/1
  Dilation/1 -> BoxForeground/1, Blob Analysis/1, Manual Switch/2
  Manual Switch/1 -> fgB/1
  BoxForeground/1 -> Manual Switch/1

== system FlameAnalysis/Background Estimator/Decomposing Red Movement/BG1/Motion Based Background Estimator/Motion Based Background Estimator/BG_running/N-Sample Enable3 ==
  Constant : Constant  OutDataTypeStr=boolean
  Constant1 : Constant  Value=0  OutDataTypeStr=boolean
  Counter Limited : simulink/Sources/Counter Limited  uplimit=sample  tsamp=-1
  Enabled Subsystem : Subsystem  TreatAsAtomicUnit=on
  Switch : Switch  Threshold=sample
  Enable : Outport
  wires:
  Counter Limited/1 -> Switch/2
  Constant1/1 -> Switch/3
  Constant/1 -> Switch/1
  Switch/1 -> Enabled Subsystem/Enable
  Enabled Subsystem/1(Out1) -> Enable/1

== system FlameAnalysis/Background Estimator/Decomposing Red Movement/BG1/Temporal Median/Temporal Median/N-Sample Enale2/Enabled Subsystem ==
  Enable : EnablePort
  Constant : Constant  Value=0  OutDataTypeStr=boolean
  Out1 : Outport  InitialOutput=1
  wires:
  Constant/1 -> Out1/1

== system FlameAnalysis/Background Estimator/Decomposing Red Movement/BG1/Temporal Median Estimator/Temporal Median Estimator/N-Sample Enale2/Enabled Subsystem ==
  Enable : EnablePort
  Constant : Constant  Value=0  OutDataTypeStr=boolean
  Out1 : Outport  InitialOutput=1
  wires:
  Constant/1 -> Out1/1

== system FlameAnalysis/Background Estimator/Decomposing Blue Movement/BG1/Motion Based Background Estimator/Motion Based Background Estimator/BG_running/N-Sample Enable3/Enabled Subsystem ==
  Enable : EnablePort
  Constant : Constant  OutDataTypeStr=boolean
  Out1 : Outport  InitialOutput=0
  wires:
  Constant/1 -> Out1/1

== system FlameAnalysis/Background Estimator/Decomposing Green Movement/BG1/Motion Based Background Estimator/Motion Based Background Estimator/BG_running/N-Sample Enable3/Enabled Subsystem ==
  Enable : EnablePort
  Constant : Constant  OutDataTypeStr=boolean
  Out1 : Outport  InitialOutput=0
  wires:
  Constant/1 -> Out1/1

== system FlameAnalysis/Background Estimator/Decomposing Red Movement/BG1/Motion Based Background Estimator/Motion Based Background Estimator/BG_running/N-Sample Enable3/Enabled Subsystem ==
  Enable : EnablePort
  Constant : Constant  OutDataTypeStr=boolean
  Out1 : Outport  InitialOutput=0
  wires:
  Constant/1 -> Out1/1

== matlab function FlameAnalysis/Flame Front Estimation/Separate Flame ==
  data: A input; y input; Flame output
function Flame = separateFlame(A,y)
[m n]=size(A);
Flame=cast(zeros([m n]),'logical');

x1=y(1);
x2=y(1)+y(3);
y1=y(2);
y2=y(2)+y(4);
if(y1>0 && y2>y1 && x1>0 && x2>x1 && y2<=m && x2<=n)
    Flame(y1:y2,x1:x2)=A(y1:y2,x1:x2);
end

== matlab function FlameAnalysis/Background Estimator/Subsystem/MATLAB Function ==
  data: J input; y output
function y = noisefiltering(J)
coder.extrinsic('medfilt2');
y=logical(zeros(size(J)));
y = logical(medfilt2(J,[3 3]));
